simulink model "Copy_3_of_proba1_poziomywsk"  (Simulink 7.0)
settings: Solver=ode1  StartTime=0.0  StopTime=Inf  FixedStep=0.001  RelTol=1e-3
PostLoadFcn:
  | ,try, rti_mdl_postloadfcn(bdroot, 'UpdateModel', 280, 'rti1005'); catch, disp(lasterr); end,
values from neighbouring files (symbols this model uses):
  Rmax = 823    [50614_9.mat]
  Rmin = 331    [50614_9.mat]
undefined symbols (not defined in the file or in its folder): sgn
libraries: simulink x68, simulink_extras x15, rtilibm x10
(part 2 of 3)

== system Copy_3_of_proba1_poziomywsk/serwomechanizmy/os1/ograniczenie1 ==
  In1 : Inport
  Compare To Constant : simulink/Logic and Bit Operations/Compare To Constant  SystemSampleTime=-1  relop=<=  const=160  LogicOutDataTypeMode=boolean  ZeroCross=off
  Compare To Constant1 : simulink/Logic and Bit Operations/Compare To Constant  SystemSampleTime=-1  relop=>=  const=-160  LogicOutDataTypeMode=boolean  ZeroCross=off
  Constant1 : Constant  Value=0
  Logical Operator : Logic  AllPortsSameDT=off  OutDataTypeMode=boolean
  Switch : Switch  Criteria=u2 ~= 0
  Out1 : Outport
  wires:
  In1/1 -> Compare To Constant/1, Compare To Constant1/1, Switch/1
  Compare To Constant1/1 -> Logical Operator/1
  Compare To Constant/1 -> Logical Operator/2
  Logical Operator/1 -> Switch/2
  Constant1/1 -> Switch/3
  Switch/1 -> Out1/1

== system Copy_3_of_proba1_poziomywsk/serwomechanizmy/os2/Position 2 ==
  Sin && Cos2 : Inport
  Reset 2 : Inport  Port=2
  Filters 2 : Subsystem
  Position Calculation 2 : Subsystem
  Out1 : Outport
  wires:
  Filters 2/1(Sin) -> Position Calculation 2/1(Sin)
  Filters 2/2(Cos) -> Position Calculation 2/2(Cos)
  Sin && Cos2/1 -> Filters 2/1(Sin && Cos)
  Reset 2/1 -> Position Calculation 2/3(Reset (Impulse))
  Position Calculation 2/1(Position) -> Out1/1

== system Copy_3_of_proba1_poziomywsk/serwomechanizmy/os2/blok bazowania ==
  bazowanie : Inport
  stop : Inport  Port=2
  DS2201IN_B1 : rtilibm/DS2201/DS2201IN_B1  SystemSampleTime=-1  BoardNo=1  ChannelNos=2  DialogFcn=gui2201in  UnitName={ 'DS2201IN_B' }  UnitValues={ 1 }  DSProperties=struct('RTI',struct('Version',uint32(1),'BlockType',struct('isSLSource',uint8(1),'isSLSink',uint8(0),'isHWSource',uint8(1),'isHWSink',uint8(0),'isSetup',uint8(0),'isInline',uint8(1),'isNonInline',uint8(0),'isInterrupt',uint8(0),'isChannelwise',uint8(0)),'IOBoardType','DS2201','UnitType','BIT','Identifier','BITIN','DialogType','ML','BlockSet','NONE','SlaveProcessor','NONE'))
  Logical Operator : Logic  Operator=OR  AllPortsSameDT=off
  S-R Flip-Flop : simulink_extras/Flip Flops/S-R Flip-Flop  SystemSampleTime=-1  initial_condition=0
  zerowanie : Subsystem  TreatAsAtomicUnit=on
  reset : Outport
  bool : Outport  Port=2
  wires:
  bazowanie/1 -> S-R Flip-Flop/1
  S-R Flip-Flop/1 -> bool/1, zerowanie/Enable
  S-R Flip-Flop/2 -> reset/1
  stop/1 -> Logical Operator/2
  Logical Operator/1 -> S-R Flip-Flop/2
  DS2201IN_B1/1 -> Logical Operator/1

== system Copy_3_of_proba1_poziomywsk/serwomechanizmy/os2/blok stopu ==
  pozycja : Inport
  Trigger : TriggerPort
  Data Store Write : DataStoreWrite  DataStoreName=u2  SampleTime=-1
  Data Store Write1 : DataStoreWrite  DataStoreName=tmp_u2  SampleTime=-1
  wires:
  pozycja/1 -> Data Store Write/1, Data Store Write1/1

== system Copy_3_of_proba1_poziomywsk/serwomechanizmy/os2/ograniczenie2 ==
  In1 : Inport
  Compare To Constant : simulink/Logic and Bit Operations/Compare To Constant  SystemSampleTime=-1  relop=<=  const=40  LogicOutDataTypeMode=boolean  ZeroCross=off
  Compare To Constant1 : simulink/Logic and Bit Operations/Compare To Constant  SystemSampleTime=-1  relop=>=  const=-40  LogicOutDataTypeMode=boolean  ZeroCross=off
  Constant1 : Constant  Value=0
  Logical Operator : Logic  AllPortsSameDT=off  OutDataTypeMode=boolean
  Switch : Switch  Criteria=u2 ~= 0
  Out1 : Outport
  wires:
  In1/1 -> Compare To Constant/1, Compare To Constant1/1, Switch/1
  Compare To Constant1/1 -> Logical Operator/1
  Compare To Constant/1 -> Logical Operator/2
  Logical Operator/1 -> Switch/2
  Constant1/1 -> Switch/3
  Switch/1 -> Out1/1

== system Copy_3_of_proba1_poziomywsk/serwomechanizmy/os3/Position 3 ==
  Sin && Cos3 : Inport
  Reset 3 : Inport  Port=2
  Filters 3 : Subsystem
  Position Calculation 3 : Subsystem
  Out1 : Outport
  wires:
  Filters 3/1(Sin) -> Position Calculation 3/1(Sin)
  Filters 3/2(Cos) -> Position Calculation 3/2(Cos)
  Sin && Cos3/1 -> Filters 3/1(Sin && Cos)
  Reset 3/1 -> Position Calculation 3/3(Reset (Impulse))
  Position Calculation 3/1(Position) -> Out1/1

== system Copy_3_of_proba1_poziomywsk/serwomechanizmy/os3/blok bazowania ==
  bazowanie : Inport
  stop : Inport  Port=2
  DS2201IN_B1 : rtilibm/DS2201/DS2201IN_B1  SystemSampleTime=-1  BoardNo=1  ChannelNos=3  DialogFcn=gui2201in  UnitName={ 'DS2201IN_B' }  UnitValues={ 1 }  DSProperties=struct('RTI',struct('Version',uint32(1),'BlockType',struct('isSLSource',uint8(1),'isSLSink',uint8(0),'isHWSource',uint8(1),'isHWSink',uint8(0),'isSetup',uint8(0),'isInline',uint8(1),'isNonInline',uint8(0),'isInterrupt',uint8(0),'isChannelwise',uint8(0)),'IOBoardType','DS2201','UnitType','BIT','Identifier','BITIN','DialogType','ML','BlockSet','NONE','SlaveProcessor','NONE'))
  Logical Operator : Logic  Operator=OR  AllPortsSameDT=off
  S-R Flip-Flop : simulink_extras/Flip Flops/S-R Flip-Flop  SystemSampleTime=-1  initial_condition=0
  zerowanie : Subsystem  TreatAsAtomicUnit=on
  reset : Outport
  bool : Outport  Port=2
  wires:
  bazowanie/1 -> S-R Flip-Flop/1
  S-R Flip-Flop/1 -> bool/1, zerowanie/Enable
  S-R Flip-Flop/2 -> reset/1
  stop/1 -> Logical Operator/2
  DS2201IN_B1/1 -> Logical Operator/1
  Logical Operator/1 -> S-R Flip-Flop/2

== system Copy_3_of_proba1_poziomywsk/serwomechanizmy/os3/blok stopu ==
  pozycja : Inport
  Trigger : TriggerPort
  Data Store Write : DataStoreWrite  DataStoreName=u3  SampleTime=-1
  Data Store Write1 : DataStoreWrite  DataStoreName=tmp_u3  SampleTime=-1
  wires:
  pozycja/1 -> Data Store Write/1, Data Store Write1/1

== system Copy_3_of_proba1_poziomywsk/serwomechanizmy/os3/ograniczenie3 ==
  In1 : Inport
  Compare To Constant : simulink/Logic and Bit Operations/Compare To Constant  SystemSampleTime=-1  relop=<=  const=40  LogicOutDataTypeMode=boolean  ZeroCross=off
  Compare To Constant1 : simulink/Logic and Bit Operations/Compare To Constant  SystemSampleTime=-1  relop=>=  const=-25  LogicOutDataTypeMode=boolean  ZeroCross=off
  Constant1 : Constant  Value=0
  Logical Operator : Logic  AllPortsSameDT=off  OutDataTypeMode=boolean
  Switch : Switch  Criteria=u2 ~= 0
  Out1 : Outport
  wires:
  In1/1 -> Compare To Constant/1, Compare To Constant1/1, Switch/1
  Compare To Constant1/1 -> Logical Operator/1
  Compare To Constant/1 -> Logical Operator/2
  Logical Operator/1 -> Switch/2
  Constant1/1 -> Switch/3
  Switch/1 -> Out1/1

== system Copy_3_of_proba1_poziomywsk/serwomechanizmy/os4/Position 4 ==
  Sin && Cos4 : Inport
  Reset 4 : Inport  Port=2
  Filters 4 : Subsystem
  Position Calculation 4 : Subsystem
  Out1 : Outport
  wires:
  Position Calculation 4/1(Position) -> Out1/1
  Reset 4/1 -> Position Calculation 4/3(Reset (Impulse))
  Sin && Cos4/1 -> Filters 4/1(Sin && Cos)
  Filters 4/2(Cos) -> Position Calculation 4/2(Cos)
  Filters 4/1(Sin) -> Position Calculation 4/1(Sin)

== system Copy_3_of_proba1_poziomywsk/serwomechanizmy/os4/blok bazowania ==
  bazowanie : Inport
  stop : Inport  Port=2
  DS2201IN_B1 : rtilibm/DS2201/DS2201IN_B1  SystemSampleTime=-1  BoardNo=1  ChannelNos=4  DialogFcn=gui2201in  UnitName={ 'DS2201IN_B' }  UnitValues={ 1 }  DSProperties=struct('RTI',struct('Version',uint32(1),'BlockType',struct('isSLSource',uint8(1),'isSLSink',uint8(0),'isHWSource',uint8(1),'isHWSink',uint8(0),'isSetup',uint8(0),'isInline',uint8(1),'isNonInline',uint8(0),'isInterrupt',uint8(0),'isChannelwise',uint8(0)),'IOBoardType','DS2201','UnitType','BIT','Identifier','BITIN','DialogType','ML','BlockSet','NONE','SlaveProcessor','NONE'))
  Logical Operator : Logic  Operator=OR  AllPortsSameDT=off
  S-R Flip-Flop : simulink_extras/Flip Flops/S-R Flip-Flop  SystemSampleTime=-1  initial_condition=0
  zerowanie : Subsystem  TreatAsAtomicUnit=on
  reset : Outport
  bool : Outport  Port=2
  wires:
  bazowanie/1 -> S-R Flip-Flop/1
  S-R Flip-Flop/1 -> bool/1, zerowanie/Enable
  S-R Flip-Flop/2 -> reset/1
  stop/1 -> Logical Operator/2
  DS2201IN_B1/1 -> Logical Operator/1
  Logical Operator/1 -> S-R Flip-Flop/2

== system Copy_3_of_proba1_poziomywsk/serwomechanizmy/os4/blok stopu ==
  pozycja : Inport
  Trigger : TriggerPort
  Data Store Write : DataStoreWrite  DataStoreName=u4  SampleTime=-1
  Data Store Write1 : DataStoreWrite  DataStoreName=tmp_u4  SampleTime=-1
  wires:
  pozycja/1 -> Data Store Write/1, Data Store Write1/1

== system Copy_3_of_proba1_poziomywsk/serwomechanizmy/os4/ograniczenie3 ==
  In1 : Inport
  Compare To Constant : simulink/Logic and Bit Operations/Compare To Constant  SystemSampleTime=-1  relop=<=  const=120  LogicOutDataTypeMode=boolean  ZeroCross=off
  Compare To Constant1 : simulink/Logic and Bit Operations/Compare To Constant  SystemSampleTime=-1  relop=>=  const=-25  LogicOutDataTypeMode=boolean  ZeroCross=off
  Constant1 : Constant  Value=0
  Logical Operator : Logic  AllPortsSameDT=off  OutDataTypeMode=boolean
  Switch : Switch  Criteria=u2 ~= 0
  Out1 : Outport
  wires:
  In1/1 -> Compare To Constant/1, Compare To Constant1/1, Switch/1
  Compare To Constant1/1 -> Logical Operator/1
  Compare To Constant/1 -> Logical Operator/2
  Logical Operator/1 -> Switch/2
  Constant1/1 -> Switch/3
  Switch/1 -> Out1/1

== system Copy_3_of_proba1_poziomywsk/serwomechanizmy/os5/Position 5 ==
  Sin && Cos5 : Inport
  Reset 5 : Inport  Port=2
  Filters 5 : Subsystem
  Position Calculation 5 : Subsystem
  Out1 : Outport
  wires:
  Position Calculation 5/1(Position) -> Out1/1
  Reset 5/1 -> Position Calculation 5/3(Reset (Impulse))
  Sin && Cos5/1 -> Filters 5/1(Sin && Cos)
  Filters 5/2(Cos) -> Position Calculation 5/2(Cos)
  Filters 5/1(Sin) -> Position Calculation 5/1(Sin)

== system Copy_3_of_proba1_poziomywsk/serwomechanizmy/os5/blok bazowania ==
  bazowanie : Inport
  stop : Inport  Port=2
  DS2201IN_B1 : rtilibm/DS2201/DS2201IN_B1  SystemSampleTime=-1  BoardNo=1  ChannelNos=5  DialogFcn=gui2201in  UnitName={ 'DS2201IN_B' }  UnitValues={ 1 }  DSProperties=struct('RTI',struct('Version',uint32(1),'BlockType',struct('isSLSource',uint8(1),'isSLSink',uint8(0),'isHWSource',uint8(1),'isHWSink',uint8(0),'isSetup',uint8(0),'isInline',uint8(1),'isNonInline',uint8(0),'isInterrupt',uint8(0),'isChannelwise',uint8(0)),'IOBoardType','DS2201','UnitType','BIT','Identifier','BITIN','DialogType','ML','BlockSet','NONE','SlaveProcessor','NONE'))
  Logical Operator : Logic  Operator=OR  AllPortsSameDT=off
  S-R Flip-Flop : simulink_extras/Flip Flops/S-R Flip-Flop  SystemSampleTime=-1  initial_condition=0
  zerowanie : Subsystem  TreatAsAtomicUnit=on
  reset : Outport
  bool : Outport  Port=2
  wires:
  bazowanie/1 -> S-R Flip-Flop/1
  S-R Flip-Flop/1 -> bool/1, zerowanie/Enable
  S-R Flip-Flop/2 -> reset/1
  stop/1 -> Logical Operator/2
  DS2201IN_B1/1 -> Logical Operator/1
  Logical Operator/1 -> S-R Flip-Flop/2

== system Copy_3_of_proba1_poziomywsk/serwomechanizmy/os5/blok stopu ==
  pozycja : Inport
  Trigger : TriggerPort
  Data Store Write : DataStoreWrite  DataStoreName=u5  SampleTime=-1
  Data Store Write1 : DataStoreWrite  DataStoreName=tmp_u5  SampleTime=-1
  wires:
  pozycja/1 -> Data Store Write/1, Data Store Write1/1

== system Copy_3_of_proba1_poziomywsk/serwomechanizmy/os5/ograniczenie3 ==
  In1 : Inport
  Compare To Constant : simulink/Logic and Bit Operations/Compare To Constant  SystemSampleTime=-1  relop=<=  const=150  LogicOutDataTypeMode=boolean  ZeroCross=off
  Compare To Constant1 : simulink/Logic and Bit Operations/Compare To Constant  SystemSampleTime=-1  relop=>=  const=-25  LogicOutDataTypeMode=boolean  ZeroCross=off
  Constant1 : Constant  Value=0
  Logical Operator : Logic  AllPortsSameDT=off  OutDataTypeMode=boolean
  Switch : Switch  Criteria=u2 ~= 0
  Out1 : Outport
  wires:
  In1/1 -> Compare To Constant/1, Compare To Constant1/1, Switch/1
  Compare To Constant1/1 -> Logical Operator/1
  Compare To Constant/1 -> Logical Operator/2
  Logical Operator/1 -> Switch/2
  Constant1/1 -> Switch/3
  Switch/1 -> Out1/1

== system Copy_3_of_proba1_poziomywsk/serwomechanizmy/os6/blok bazowania ==
  bazowanie : Inport
  stop : Inport  Port=2
  DS2201IN_B1 : rtilibm/DS2201/DS2201IN_B1  SystemSampleTime=-1  BoardNo=1  ChannelNos=6  DialogFcn=gui2201in  UnitName={ 'DS2201IN_B' }  UnitValues={ 1 }  DSProperties=struct('RTI',struct('Version',uint32(1),'BlockType',struct('isSLSource',uint8(1),'isSLSink',uint8(0),'isHWSource',uint8(1),'isHWSink',uint8(0),'isSetup',uint8(0),'isInline',uint8(1),'isNonInline',uint8(0),'isInterrupt',uint8(0),'isChannelwise',uint8(0)),'IOBoardType','DS2201','UnitType','BIT','Identifier','BITIN','DialogType','ML','BlockSet','NONE','SlaveProcessor','NONE'))
  Logical Operator : Logic  Operator=OR  AllPortsSameDT=off
  S-R Flip-Flop : simulink_extras/Flip Flops/S-R Flip-Flop  SystemSampleTime=-1  initial_condition=0
  zerowanie : Subsystem  TreatAsAtomicUnit=on
  reset : Outport
  bool : Outport  Port=2
  wires:
  bazowanie/1 -> S-R Flip-Flop/1
  S-R Flip-Flop/1 -> bool/1, zerowanie/Enable
  S-R Flip-Flop/2 -> reset/1
  stop/1 -> Logical Operator/2
  DS2201IN_B1/1 -> Logical Operator/1
  Logical Operator/1 -> S-R Flip-Flop/2

== system Copy_3_of_proba1_poziomywsk/serwomechanizmy/os6/blok stopu ==
  pozycja : Inport
  Trigger : TriggerPort
  Data Store Write : DataStoreWrite  DataStoreName=u0  SampleTime=-1
  Data Store Write1 : DataStoreWrite  DataStoreName=tmp_u0  SampleTime=-1
  wires:
  pozycja/1 -> Data Store Write/1, Data Store Write1/1

== system Copy_3_of_proba1_poziomywsk/serwomechanizmy/os6/ograniczenie3 ==
  In1 : Inport
  Compare To Constant : simulink/Logic and Bit Operations/Compare To Constant  SystemSampleTime=-1  relop=<=  const=890  LogicOutDataTypeMode=boolean  ZeroCross=off
  Compare To Constant1 : simulink/Logic and Bit Operations/Compare To Constant  SystemSampleTime=-1  relop=>=  const=0  LogicOutDataTypeMode=boolean  ZeroCross=off
  Constant1 : Constant  Value=0
  Logical Operator : Logic  AllPortsSameDT=off  OutDataTypeMode=boolean
  Switch : Switch  Criteria=u2 ~= 0
  Out1 : Outport
  wires:
  In1/1 -> Compare To Constant/1, Compare To Constant1/1, Switch/1
  Compare To Constant1/1 -> Logical Operator/1
  Compare To Constant/1 -> Logical Operator/2
  Logical Operator/1 -> Switch/2
  Constant1/1 -> Switch/3
  Switch/1 -> Out1/1

== system Copy_3_of_proba1_poziomywsk/serwomechanizmy/os6/skalowanie ==
  In1 : Inport
  Fcn : Fcn  Expr=(u(1)*(2^23)*pi())/1000
  Gain2 : Gain  Gain=1.25/pi()
  Out1 : Outport
  wires:
  Fcn/1 -> Gain2/1
  Gain2/1 -> Out1/1
  In1/1 -> Fcn/1

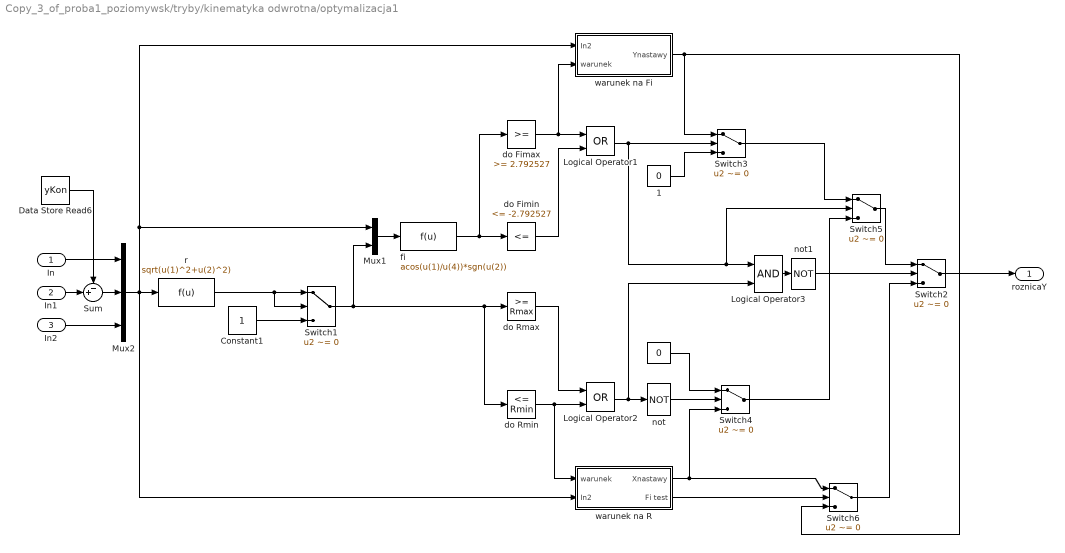
== system Copy_3_of_proba1_poziomywsk/tryby/kinematyka odwrotna/optymalizacja1 ==
  In : Inport
  In1 : Inport  Port=2
  In2 : Inport  Port=3
  " " : Constant  Value=0  OutDataTypeMode=double
  " 1" : Constant  Value=0  OutDataTypeMode=double
  Constant1 : Constant  OutDataTypeMode=double
  Data Store Read6 : DataStoreRead  DataStoreName=yKon  SampleTime=0
  Logical Operator1 : Logic  Operator=OR  AllPortsSameDT=off  OutDataTypeMode=boolean
  Logical Operator2 : Logic  Operator=OR  AllPortsSameDT=off  OutDataTypeMode=boolean
  Logical Operator3 : Logic  AllPortsSameDT=off  OutDataTypeMode=boolean
  Mux1 : Mux  Inputs=2
  Mux2 : Mux  Inputs=3
  Sum : Sum  Inputs=-+|
  Switch1 : Switch  Criteria=u2 ~= 0  OutDataTypeMode=double
  Switch{2..6} (5 alike) : Switch  Criteria=u2 ~= 0
  do Fimax : simulink/Logic and Bit Operations/Compare To Constant  SystemSampleTime=-1  relop=>=  const=2.792527  LogicOutDataTypeMode=uint8  ZeroCross=off
  do Fimin : simulink/Logic and Bit Operations/Compare To Constant  SystemSampleTime=-1  relop=<=  const=-2.792527  LogicOutDataTypeMode=uint8  ZeroCross=off
  do Rmax : simulink/Logic and Bit Operations/Compare To Constant  SystemSampleTime=-1  relop=>=  const=Rmax  LogicOutDataTypeMode=uint8  ZeroCross=off
  do Rmin : simulink/Logic and Bit Operations/Compare To Constant  SystemSampleTime=-1  relop=<=  const=Rmin  LogicOutDataTypeMode=uint8  ZeroCross=off
  fi : Fcn  Expr=acos(u(1)/u(4))*sgn(u(2))
  not : Logic  Operator=NOT  AllPortsSameDT=off  OutDataTypeMode=boolean
  not1 : Logic  Operator=NOT  AllPortsSameDT=off  OutDataTypeMode=boolean
  r : Fcn  Expr=sqrt(u(1)^2+u(2)^2)
  warunek na Fi : Subsystem  TreatAsAtomicUnit=on
  warunek na R : Subsystem  TreatAsAtomicUnit=on
  roznicaY : Outport
  wires:
  Switch6/1 -> Switch2/3
  warunek na R/2(Fi test) -> Switch6/2
  not1/1 -> Switch2/2
  Switch3/1 -> Switch5/1
  Switch4/1 -> Switch5/3
  Switch5/1 -> Switch2/1
  Logical Operator3/1 -> not1/1
  " 1"/1 -> Switch3/3
  " "/1 -> Switch4/1
  not/1 -> Switch4/2
  warunek na R/1(Xnastawy) -> Switch4/3, Switch6/1
  warunek na Fi/1(Ynastawy) -> Switch3/1, Switch6/3
  Logical Operator1/1 -> Switch3/2, Logical Operator3/1, Switch5/2
  Logical Operator2/1 -> not/1, Logical Operator3/2
  do Rmin/1 -> Logical Operator2/2, warunek na R/1(warunek)
  do Rmax/1 -> Logical Operator2/1
  do Fimin/1 -> Logical Operator1/2
  do Fimax/1 -> warunek na Fi/2(warunek), Logical Operator1/1
  fi/1 -> do Fimin/1, do Fimax/1
  Constant1/1 -> Switch1/3
  Mux1/1 -> fi/1
  Switch1/1 -> Mux1/2, do Rmax/1, do Rmin/1
  r/1 -> Switch1/2, Switch1/1
  Mux2/1 -> r/1, Mux1/1, warunek na Fi/1(In2), warunek na R/2(In2)
  In/1 -> Mux2/1
  In2/1 -> Mux2/3
  Switch2/1 -> roznicaY/1
  Sum/1 -> Mux2/2
  In1/1 -> Sum/2
  Data Store Read6/1 -> Sum/1

== system Copy_3_of_proba1_poziomywsk/tryby/kinematyka odwrotna/podaj wyliczone wartosci ==
  obliczoneFi1 : Inport
  obliczoneFi2 : Inport  Port=2
  obliczoneFi3 : Inport  Port=3
  obliczoneDist : Inport  Port=4
  Enable : EnablePort
  Data Store Write : DataStoreWrite  DataStoreName=obliczoneFi1  SampleTime=-1
  Data Store Write1 : DataStoreWrite  DataStoreName=obliczoneFi2  SampleTime=-1
  Data Store Write2 : DataStoreWrite  DataStoreName=obliczoneFi3  SampleTime=-1
  Data Store Write3 : DataStoreWrite  DataStoreName=obliczoneDist  SampleTime=-1
  wires:
  obliczoneFi1/1 -> Data Store Write/1
  obliczoneFi2/1 -> Data Store Write1/1
  obliczoneFi3/1 -> Data Store Write2/1
  obliczoneDist/1 -> Data Store Write3/1

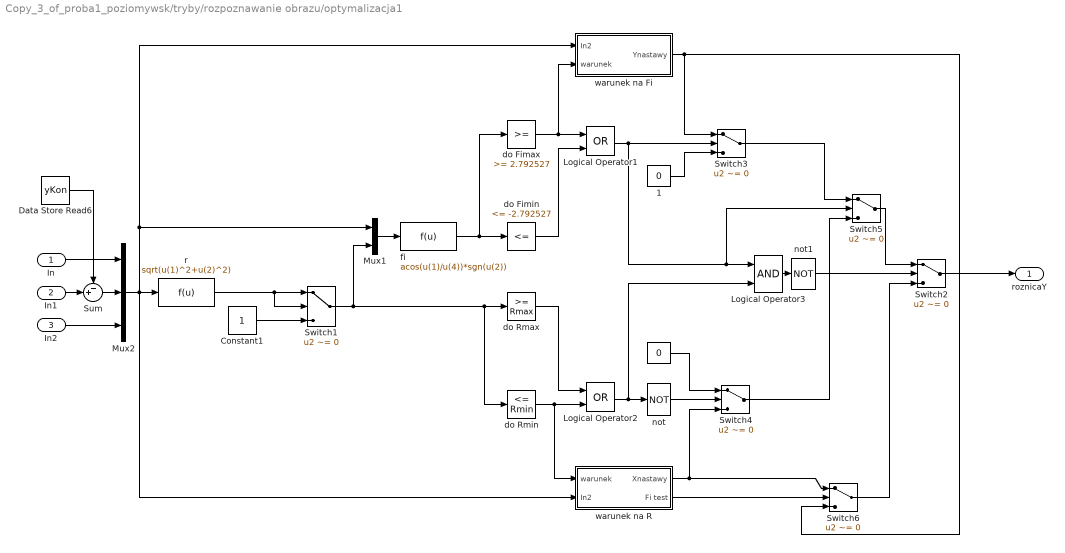
== system Copy_3_of_proba1_poziomywsk/tryby/rozpoznawanie obrazu/optymalizacja1 ==
  In : Inport
  In1 : Inport  Port=2
  In2 : Inport  Port=3
  " " : Constant  Value=0  OutDataTypeMode=double
  " 1" : Constant  Value=0  OutDataTypeMode=double
  Constant1 : Constant  OutDataTypeMode=double
  Data Store Read6 : DataStoreRead  DataStoreName=yKon  SampleTime=-1
  Logical Operator1 : Logic  Operator=OR  AllPortsSameDT=off  OutDataTypeMode=boolean
  Logical Operator2 : Logic  Operator=OR  AllPortsSameDT=off  OutDataTypeMode=boolean
  Logical Operator3 : Logic  AllPortsSameDT=off  OutDataTypeMode=boolean
  Mux1 : Mux  Inputs=2
  Mux2 : Mux  Inputs=3
  Sum : Sum  Inputs=-+|
  Switch1 : Switch  Criteria=u2 ~= 0  OutDataTypeMode=double
  Switch{2..6} (5 alike) : Switch  Criteria=u2 ~= 0
  do Fimax : simulink/Logic and Bit Operations/Compare To Constant  SystemSampleTime=-1  relop=>=  const=2.792527  LogicOutDataTypeMode=uint8  ZeroCross=off
  do Fimin : simulink/Logic and Bit Operations/Compare To Constant  SystemSampleTime=-1  relop=<=  const=-2.792527  LogicOutDataTypeMode=uint8  ZeroCross=off
  do Rmax : simulink/Logic and Bit Operations/Compare To Constant  SystemSampleTime=-1  relop=>=  const=Rmax  LogicOutDataTypeMode=uint8  ZeroCross=off
  do Rmin : simulink/Logic and Bit Operations/Compare To Constant  SystemSampleTime=-1  relop=<=  const=Rmin  LogicOutDataTypeMode=uint8  ZeroCross=off
  fi : Fcn  Expr=acos(u(1)/u(4))*sgn(u(2))
  not : Logic  Operator=NOT  AllPortsSameDT=off  OutDataTypeMode=boolean
  not1 : Logic  Operator=NOT  AllPortsSameDT=off  OutDataTypeMode=boolean
  r : Fcn  Expr=sqrt(u(1)^2+u(2)^2)
  warunek na Fi : Subsystem  TreatAsAtomicUnit=on
  warunek na R : Subsystem  TreatAsAtomicUnit=on
  roznicaY : Outport
  wires:
  Data Store Read6/1 -> Sum/1
  In1/1 -> Sum/2
  Sum/1 -> Mux2/2
  Switch2/1 -> roznicaY/1
  In2/1 -> Mux2/3
  In/1 -> Mux2/1
  Mux2/1 -> warunek na R/2(In2), warunek na Fi/1(In2), Mux1/1, r/1
  r/1 -> Switch1/1, Switch1/2
  Switch1/1 -> do Rmin/1, do Rmax/1, Mux1/2
  Mux1/1 -> fi/1
  Constant1/1 -> Switch1/3
  fi/1 -> do Fimax/1, do Fimin/1
  do Fimax/1 -> Logical Operator1/1, warunek na Fi/2(warunek)
  do Fimin/1 -> Logical Operator1/2
  do Rmax/1 -> Logical Operator2/1
  do Rmin/1 -> warunek na R/1(warunek), Logical Operator2/2
  Logical Operator2/1 -> Logical Operator3/2, not/1
  Logical Operator1/1 -> Switch5/2, Logical Operator3/1, Switch3/2
  warunek na Fi/1(Ynastawy) -> Switch6/3, Switch3/1
  warunek na R/1(Xnastawy) -> Switch6/1, Switch4/3
  not/1 -> Switch4/2
  " "/1 -> Switch4/1
  " 1"/1 -> Switch3/3
  Logical Operator3/1 -> not1/1
  Switch5/1 -> Switch2/1
  Switch4/1 -> Switch5/3
  Switch3/1 -> Switch5/1
  not1/1 -> Switch2/2
  warunek na R/2(Fi test) -> Switch6/2
  Switch6/1 -> Switch2/3

== system Copy_3_of_proba1_poziomywsk/tryby/rozpoznawanie obrazu/podaj wyliczone wartosci ==
  obliczoneFi1 : Inport
  obliczoneFi2 : Inport  Port=2
  obliczoneFi3 : Inport  Port=3
  obliczoneDist : Inport  Port=4
  Enable : EnablePort
  Data Store Write : DataStoreWrite  DataStoreName=obliczoneFi1  SampleTime=-1
  Data Store Write1 : DataStoreWrite  DataStoreName=obliczoneFi2  SampleTime=-1
  Data Store Write2 : DataStoreWrite  DataStoreName=obliczoneFi3  SampleTime=-1
  Data Store Write3 : DataStoreWrite  DataStoreName=obliczoneDist  SampleTime=-1
  wires:
  obliczoneDist/1 -> Data Store Write3/1
  obliczoneFi3/1 -> Data Store Write2/1
  obliczoneFi2/1 -> Data Store Write1/1
  obliczoneFi1/1 -> Data Store Write/1

== system Copy_3_of_proba1_poziomywsk/RTI Data/RTI Data Store/RTI Data Store/RTI Data Store ==
  RTI Data Store : Subsystem
      mask Type: RTI_DATA_STORE
      mask Description:
      | RTI Data Store Block. This block is used by RTI to store internal model dependent data. Deleting this block will result in data loss.
      | 
      | NEVER DELETE, COPY, OR MODIFY THIS BLOCK!
      mask Help:
      | RTI Data Store Block. This block is used by RTI to store internal model dependent data. Deleting this block will result in data loss.
      | 
      | NEVER DELETE, COPY, OR MODIFY THIS BLOCK!
      mask Display: text(0.5, 0.5, ' ', 'HorizontalAlignment', 'center');

== system Copy_3_of_proba1_poziomywsk/serwomechanizmy/os1/Position 1/Filters 1 ==
  Sin && Cos : Inport
  Analog Butterworth LP Filter : Subsystem  mask(buttap){@1=2*pi*16, @2=1}
      mask prompts: @1 "Cutoff frequency (rad/sec)"; @2 "Order"
      mask help:
      | Analog Butterworth low pass filter.
      |
      | (Requires Signal Processing Toolbox)
      mask init:
      | [z,p,k]=buttap(@2); z=@1*z; p=@1*p; k=real(prod(-p)); [num,den]=zp2tf(z,p,k); w=logspace(log10(@1/10),log10(10*@1),20); h=freqs(num,den,w);
      mask Help: Butterworth low pass filter using MATLAB's butter command.
      mask Display: plot(20*log10(w),20*log10(abs(h)))
  Analog Butterworth LP Filter1 : Subsystem  mask(buttap){@1=2*pi*16, @2=1}
      mask prompts: @1 "Cutoff frequency (rad/sec)"; @2 "Order"
      mask help:
      | Analog Butterworth low pass filter.
      |
      | (Requires Signal Processing Toolbox)
      mask init:
      | [z,p,k]=buttap(@2); z=@1*z; p=@1*p; k=real(prod(-p)); [num,den]=zp2tf(z,p,k); w=logspace(log10(@1/10),log10(10*@1),20); h=freqs(num,den,w);
      mask Help: Butterworth low pass filter using MATLAB's butter command.
      mask Display: plot(20*log10(w),20*log10(abs(h)))
  Demux : Demux  Outputs=2
  Sin : Outport
  Cos : Outport  Port=2
  wires:
  Demux/2 -> Analog Butterworth LP Filter1/1(In1)
  Demux/1 -> Analog Butterworth LP Filter/1(In1)
  Sin && Cos/1 -> Demux/1
  Analog Butterworth LP Filter1/1(Out1) -> Cos/1
  Analog Butterworth LP Filter/1(Out1) -> Sin/1

== system Copy_3_of_proba1_poziomywsk/serwomechanizmy/os1/Position 1/Position Calculation 1 ==
  Sin : Inport
  Cos : Inport  Port=2
  Reset (Impulse) : Inport  Port=3
  Atan2 : Fcn  Expr=atan2(u[1],u[2])
  Conversion Rad to Deg : Gain  Gain=180/pi  SaturateOnIntegerOverflow=on
  Conversion Rotation to Angle : Gain  Gain=2*pi  SaturateOnIntegerOverflow=on
  Dead Zone : DeadZone  LowerValue=-5000  UpperValue=5000  SaturateOnIntegerOverflow=on
  Derivative : Derivative
  Gear : Gain  Gain=6.33e-3  SaturateOnIntegerOverflow=on
  Init Angle : Switch  Threshold=1  SaturateOnIntegerOverflow=on  InputSameDT=on
  Memory : Memory  Orientation=left
  Memory1 : Memory  Orientation=left
  Mux : Mux  Inputs=2
  Product : Product  SaturateOnIntegerOverflow=on  RndMeth=Zero  InputSameDT=on
  Saturation : Saturate  UpperLimit=1  LowerLimit=-1
  Sum : Sum  Inputs=+-  SaturateOnIntegerOverflow=on  InputSameDT=on
  Sum1 : Sum  Inputs=++-  SaturateOnIntegerOverflow=on  InputSameDT=on
  Position : Outport
  wires:
  Init Angle/1 -> Memory1/1, Sum1/3
  Memory1/1 -> Init Angle/1
  Product/1 -> Memory/1, Conversion Rotation to Angle/1
  Memory/1 -> Sum/1
  Cos/1 -> Mux/2
  Atan2/1 -> Init Angle/3, Sum1/2, Derivative/1
  Reset (Impulse)/1 -> Init Angle/2, Product/2
  Conversion Rotation to Angle/1 -> Sum1/1
  Saturation/1 -> Sum/2
  Conversion Rad to Deg/1 -> Position/1
  Sin/1 -> Mux/1
  Mux/1 -> Atan2/1
  Derivative/1 -> Dead Zone/1
  Dead Zone/1 -> Saturation/1
  Sum/1 -> Product/1
  Sum1/1 -> Gear/1
  Gear/1 -> Conversion Rad to Deg/1

== system Copy_3_of_proba1_poziomywsk/serwomechanizmy/os1/blok bazowania/zerowanie ==
  Enable : EnablePort
  Constant : Constant  Value=0
  Data Store Write : DataStoreWrite  DataStoreName=u1  SampleTime=-1
  Data Store Write1 : DataStoreWrite  DataStoreName=tmp_u1  SampleTime=-1
  wires:
  Constant/1 -> Data Store Write/1, Data Store Write1/1

== system Copy_3_of_proba1_poziomywsk/serwomechanizmy/os2/Position 2/Filters 2 ==
  Sin && Cos : Inport
  Analog Butterworth LP Filter : Subsystem  mask(buttap){@1=2*pi*16, @2=1}
      mask prompts: @1 "Cutoff frequency (rad/sec)"; @2 "Order"
      mask help:
      | Analog Butterworth low pass filter.
      |
      | (Requires Signal Processing Toolbox)
      mask init:
      | [z,p,k]=buttap(@2); z=@1*z; p=@1*p; k=real(prod(-p)); [num,den]=zp2tf(z,p,k); w=logspace(log10(@1/10),log10(10*@1),20); h=freqs(num,den,w);
      mask Help: Butterworth low pass filter using MATLAB's butter command.
      mask Display: plot(20*log10(w),20*log10(abs(h)))
  Analog Butterworth LP Filter1 : Subsystem  mask(buttap){@1=2*pi*16, @2=1}
      mask prompts: @1 "Cutoff frequency (rad/sec)"; @2 "Order"
      mask help:
      | Analog Butterworth low pass filter.
      |
      | (Requires Signal Processing Toolbox)
      mask init:
      | [z,p,k]=buttap(@2); z=@1*z; p=@1*p; k=real(prod(-p)); [num,den]=zp2tf(z,p,k); w=logspace(log10(@1/10),log10(10*@1),20); h=freqs(num,den,w);
      mask Help: Butterworth low pass filter using MATLAB's butter command.
      mask Display: plot(20*log10(w),20*log10(abs(h)))
  Demux : Demux  Outputs=2
  Sin : Outport
  Cos : Outport  Port=2
  wires:
  Demux/2 -> Analog Butterworth LP Filter1/1(In1)
  Demux/1 -> Analog Butterworth LP Filter/1(In1)
  Sin && Cos/1 -> Demux/1
  Analog Butterworth LP Filter1/1(Out1) -> Cos/1
  Analog Butterworth LP Filter/1(Out1) -> Sin/1

== system Copy_3_of_proba1_poziomywsk/serwomechanizmy/os2/Position 2/Position Calculation 2 ==
  Sin : Inport
  Cos : Inport  Port=2
  Reset (Impulse) : Inport  Port=3
  Atan2 : Fcn  Expr=atan2(u[1],u[2])
  Conversion Rad to Deg : Gain  Gain=180/pi  SaturateOnIntegerOverflow=on
  Conversion Rotation to Angle : Gain  Gain=2*pi  SaturateOnIntegerOverflow=on
  Dead Zone : DeadZone  LowerValue=-5000  UpperValue=5000  SaturateOnIntegerOverflow=on
  Derivative : Derivative
  Gear : Gain  Gain=6.37e-3  SaturateOnIntegerOverflow=on
  Init Angle : Switch  Threshold=1  SaturateOnIntegerOverflow=on  InputSameDT=on
  Memory : Memory  Orientation=left
  Memory1 : Memory  Orientation=left
  Mux : Mux  Inputs=2
  Product : Product  SaturateOnIntegerOverflow=on  RndMeth=Zero  InputSameDT=on
  Saturation : Saturate  UpperLimit=1  LowerLimit=-1
  Sum : Sum  Inputs=+-  SaturateOnIntegerOverflow=on  InputSameDT=on
  Sum1 : Sum  Inputs=++-  SaturateOnIntegerOverflow=on  InputSameDT=on
  Position : Outport
  wires:
  Init Angle/1 -> Memory1/1, Sum1/3
  Memory1/1 -> Init Angle/1
  Product/1 -> Memory/1, Conversion Rotation to Angle/1
  Memory/1 -> Sum/1
  Cos/1 -> Mux/2
  Atan2/1 -> Init Angle/3, Sum1/2, Derivative/1
  Reset (Impulse)/1 -> Init Angle/2, Product/2
  Conversion Rotation to Angle/1 -> Sum1/1
  Saturation/1 -> Sum/2
  Conversion Rad to Deg/1 -> Position/1
  Sin/1 -> Mux/1
  Mux/1 -> Atan2/1
  Derivative/1 -> Dead Zone/1
  Dead Zone/1 -> Saturation/1
  Sum/1 -> Product/1
  Sum1/1 -> Gear/1
  Gear/1 -> Conversion Rad to Deg/1

== system Copy_3_of_proba1_poziomywsk/serwomechanizmy/os2/blok bazowania/zerowanie ==
  Enable : EnablePort
  Constant : Constant  Value=0
  Data Store Write : DataStoreWrite  DataStoreName=u2  SampleTime=-1
  Data Store Write1 : DataStoreWrite  DataStoreName=tmp_u2  SampleTime=-1
  wires:
  Constant/1 -> Data Store Write/1, Data Store Write1/1

== system Copy_3_of_proba1_poziomywsk/serwomechanizmy/os3/Position 3/Filters 3 ==
  Sin && Cos : Inport
  Analog Butterworth LP Filter : Subsystem  mask(buttap){@1=2*pi*16, @2=1}
      mask prompts: @1 "Cutoff frequency (rad/sec)"; @2 "Order"
      mask help:
      | Analog Butterworth low pass filter.
      |
      | (Requires Signal Processing Toolbox)
      mask init:
      | [z,p,k]=buttap(@2); z=@1*z; p=@1*p; k=real(prod(-p)); [num,den]=zp2tf(z,p,k); w=logspace(log10(@1/10),log10(10*@1),20); h=freqs(num,den,w);
      mask Help: Butterworth low pass filter using MATLAB's butter command.
      mask Display: plot(20*log10(w),20*log10(abs(h)))
  Analog Butterworth LP Filter1 : Subsystem  mask(buttap){@1=2*pi*16, @2=1}
      mask prompts: @1 "Cutoff frequency (rad/sec)"; @2 "Order"
      mask help:
      | Analog Butterworth low pass filter.
      |
      | (Requires Signal Processing Toolbox)
      mask init:
      | [z,p,k]=buttap(@2); z=@1*z; p=@1*p; k=real(prod(-p)); [num,den]=zp2tf(z,p,k); w=logspace(log10(@1/10),log10(10*@1),20); h=freqs(num,den,w);
      mask Help: Butterworth low pass filter using MATLAB's butter command.
      mask Display: plot(20*log10(w),20*log10(abs(h)))
  Demux : Demux  Outputs=2
  Sin : Outport
  Cos : Outport  Port=2
  wires:
  Demux/2 -> Analog Butterworth LP Filter1/1(In1)
  Demux/1 -> Analog Butterworth LP Filter/1(In1)
  Sin && Cos/1 -> Demux/1
  Analog Butterworth LP Filter1/1(Out1) -> Cos/1
  Analog Butterworth LP Filter/1(Out1) -> Sin/1

== system Copy_3_of_proba1_poziomywsk/serwomechanizmy/os3/Position 3/Position Calculation 3 ==
  Sin : Inport
  Cos : Inport  Port=2
  Reset (Impulse) : Inport  Port=3
  Atan2 : Fcn  Expr=atan2(u[1],u[2])
  Conversion Rad to Deg : Gain  Gain=180/pi  SaturateOnIntegerOverflow=on
  Conversion Rotation to Angle : Gain  Gain=2*pi  SaturateOnIntegerOverflow=on
  Dead Zone : DeadZone  LowerValue=-5000  UpperValue=5000  SaturateOnIntegerOverflow=on
  Derivative : Derivative
  Gear : Gain  Gain=6.33e-3  SaturateOnIntegerOverflow=on
  Init Angle : Switch  Threshold=1  SaturateOnIntegerOverflow=on  InputSameDT=on
  Memory : Memory  Orientation=left
  Memory1 : Memory  Orientation=left
  Mux : Mux  Inputs=2
  Product : Product  SaturateOnIntegerOverflow=on  RndMeth=Zero  InputSameDT=on
  Saturation : Saturate  UpperLimit=1  LowerLimit=-1
  Sum : Sum  Inputs=+-  SaturateOnIntegerOverflow=on  InputSameDT=on
  Sum1 : Sum  Inputs=++-  SaturateOnIntegerOverflow=on  InputSameDT=on
  Position : Outport
  wires:
  Init Angle/1 -> Memory1/1, Sum1/3
  Memory1/1 -> Init Angle/1
  Product/1 -> Memory/1, Conversion Rotation to Angle/1
  Memory/1 -> Sum/1
  Cos/1 -> Mux/2
  Atan2/1 -> Init Angle/3, Sum1/2, Derivative/1
  Reset (Impulse)/1 -> Init Angle/2, Product/2
  Conversion Rotation to Angle/1 -> Sum1/1
  Saturation/1 -> Sum/2
  Conversion Rad to Deg/1 -> Position/1
  Sin/1 -> Mux/1
  Mux/1 -> Atan2/1
  Derivative/1 -> Dead Zone/1
  Dead Zone/1 -> Saturation/1
  Sum/1 -> Product/1
  Sum1/1 -> Gear/1
  Gear/1 -> Conversion Rad to Deg/1

== system Copy_3_of_proba1_poziomywsk/serwomechanizmy/os3/blok bazowania/zerowanie ==
  Enable : EnablePort
  Constant : Constant  Value=0
  Data Store Write : DataStoreWrite  DataStoreName=u3  SampleTime=-1
  Data Store Write1 : DataStoreWrite  DataStoreName=tmp_u3  SampleTime=-1
  wires:
  Constant/1 -> Data Store Write/1, Data Store Write1/1

== system Copy_3_of_proba1_poziomywsk/serwomechanizmy/os4/Position 4/Filters 4 ==
  Sin && Cos : Inport
  Analog Butterworth LP Filter : Subsystem  mask(buttap){@1=2*pi*16, @2=1}
      mask prompts: @1 "Cutoff frequency (rad/sec)"; @2 "Order"
      mask help:
      | Analog Butterworth low pass filter.
      |
      | (Requires Signal Processing Toolbox)
      mask init:
      | [z,p,k]=buttap(@2); z=@1*z; p=@1*p; k=real(prod(-p)); [num,den]=zp2tf(z,p,k); w=logspace(log10(@1/10),log10(10*@1),20); h=freqs(num,den,w);
      mask Help: Butterworth low pass filter using MATLAB's butter command.
      mask Display: plot(20*log10(w),20*log10(abs(h)))
  Analog Butterworth LP Filter1 : Subsystem  mask(buttap){@1=2*pi*16, @2=1}
      mask prompts: @1 "Cutoff frequency (rad/sec)"; @2 "Order"
      mask help:
      | Analog Butterworth low pass filter.
      |
      | (Requires Signal Processing Toolbox)
      mask init:
      | [z,p,k]=buttap(@2); z=@1*z; p=@1*p; k=real(prod(-p)); [num,den]=zp2tf(z,p,k); w=logspace(log10(@1/10),log10(10*@1),20); h=freqs(num,den,w);
      mask Help: Butterworth low pass filter using MATLAB's butter command.
      mask Display: plot(20*log10(w),20*log10(abs(h)))
  Demux : Demux  Outputs=2
  Sin : Outport
  Cos : Outport  Port=2
  wires:
  Analog Butterworth LP Filter/1(Out1) -> Sin/1
  Analog Butterworth LP Filter1/1(Out1) -> Cos/1
  Sin && Cos/1 -> Demux/1
  Demux/1 -> Analog Butterworth LP Filter/1(In1)
  Demux/2 -> Analog Butterworth LP Filter1/1(In1)

== system Copy_3_of_proba1_poziomywsk/serwomechanizmy/os4/Position 4/Position Calculation 4 ==
  Sin : Inport
  Cos : Inport  Port=2
  Reset (Impulse) : Inport  Port=3
  Atan2 : Fcn  Expr=atan2(u[1],u[2])
  Conversion Rad to Deg : Gain  Gain=180/pi  SaturateOnIntegerOverflow=on
  Conversion Rotation to Angle : Gain  Gain=2*pi  SaturateOnIntegerOverflow=on
  Dead Zone : DeadZone  LowerValue=-5000  UpperValue=5000  SaturateOnIntegerOverflow=on
  Derivative : Derivative
  Gear : Gain  Gain=7.87e-3  SaturateOnIntegerOverflow=on
  Init Angle : Switch  Threshold=1  SaturateOnIntegerOverflow=on  InputSameDT=on
  Memory : Memory  Orientation=left
  Memory1 : Memory  Orientation=left
  Mux : Mux  Inputs=2
  Product : Product  SaturateOnIntegerOverflow=on  RndMeth=Zero  InputSameDT=on
  Saturation : Saturate  UpperLimit=1  LowerLimit=-1
  Sum : Sum  Inputs=+-  SaturateOnIntegerOverflow=on  InputSameDT=on
  Sum1 : Sum  Inputs=++-  SaturateOnIntegerOverflow=on  InputSameDT=on
  Position : Outport
  wires:
  Gear/1 -> Conversion Rad to Deg/1
  Sum1/1 -> Gear/1
  Sum/1 -> Product/1
  Dead Zone/1 -> Saturation/1
  Derivative/1 -> Dead Zone/1
  Mux/1 -> Atan2/1
  Sin/1 -> Mux/1
  Conversion Rad to Deg/1 -> Position/1
  Saturation/1 -> Sum/2
  Conversion Rotation to Angle/1 -> Sum1/1
  Reset (Impulse)/1 -> Product/2, Init Angle/2
  Atan2/1 -> Derivative/1, Sum1/2, Init Angle/3
  Cos/1 -> Mux/2
  Memory/1 -> Sum/1
  Product/1 -> Conversion Rotation to Angle/1, Memory/1
  Memory1/1 -> Init Angle/1
  Init Angle/1 -> Sum1/3, Memory1/1

== system Copy_3_of_proba1_poziomywsk/serwomechanizmy/os4/blok bazowania/zerowanie ==
  Enable : EnablePort
  Constant : Constant  Value=0
  Data Store Write : DataStoreWrite  DataStoreName=u4  SampleTime=-1
  Data Store Write1 : DataStoreWrite  DataStoreName=tmp_u4  SampleTime=-1
  wires:
  Constant/1 -> Data Store Write/1, Data Store Write1/1

== system Copy_3_of_proba1_poziomywsk/serwomechanizmy/os5/Position 5/Filters 5 ==
  Sin && Cos : Inport
  Analog Butterworth LP Filter : Subsystem  mask(buttap){@1=2*pi*16, @2=1}
      mask prompts: @1 "Cutoff frequency (rad/sec)"; @2 "Order"
      mask help:
      | Analog Butterworth low pass filter.
      |
      | (Requires Signal Processing Toolbox)
      mask init:
      | [z,p,k]=buttap(@2); z=@1*z; p=@1*p; k=real(prod(-p)); [num,den]=zp2tf(z,p,k); w=logspace(log10(@1/10),log10(10*@1),20); h=freqs(num,den,w);
      mask Help: Butterworth low pass filter using MATLAB's butter command.
      mask Display: plot(20*log10(w),20*log10(abs(h)))
  Analog Butterworth LP Filter1 : Subsystem  mask(buttap){@1=2*pi*16, @2=1}
      mask prompts: @1 "Cutoff frequency (rad/sec)"; @2 "Order"
      mask help:
      | Analog Butterworth low pass filter.
      |
      | (Requires Signal Processing Toolbox)
      mask init:
      | [z,p,k]=buttap(@2); z=@1*z; p=@1*p; k=real(prod(-p)); [num,den]=zp2tf(z,p,k); w=logspace(log10(@1/10),log10(10*@1),20); h=freqs(num,den,w);
      mask Help: Butterworth low pass filter using MATLAB's butter command.
      mask Display: plot(20*log10(w),20*log10(abs(h)))
  Demux : Demux  Outputs=2
  Sin : Outport
  Cos : Outport  Port=2
  wires:
  Analog Butterworth LP Filter/1(Out1) -> Sin/1
  Analog Butterworth LP Filter1/1(Out1) -> Cos/1
  Sin && Cos/1 -> Demux/1
  Demux/1 -> Analog Butterworth LP Filter/1(In1)
  Demux/2 -> Analog Butterworth LP Filter1/1(In1)

== system Copy_3_of_proba1_poziomywsk/serwomechanizmy/os5/Position 5/Position Calculation 5 ==
  Sin : Inport
  Cos : Inport  Port=2
  Reset (Impulse) : Inport  Port=3
  Atan2 : Fcn  Expr=atan2(u[1],u[2])
  Conversion Rad to Deg : Gain  Gain=180/pi  SaturateOnIntegerOverflow=on
  Conversion Rotation to Angle : Gain  Gain=2*pi  SaturateOnIntegerOverflow=on
  Dead Zone : DeadZone  LowerValue=-5000  UpperValue=5000  SaturateOnIntegerOverflow=on
  Derivative : Derivative
  Gear : Gain  Gain=1.32e-2  SaturateOnIntegerOverflow=on
  Init Angle : Switch  Threshold=1  SaturateOnIntegerOverflow=on  InputSameDT=on
  Memory : Memory  Orientation=left
  Memory1 : Memory  Orientation=left
  Mux : Mux  Inputs=2
  Product : Product  SaturateOnIntegerOverflow=on  RndMeth=Zero  InputSameDT=on
  Saturation : Saturate  UpperLimit=1  LowerLimit=-1
  Sum : Sum  Inputs=+-  SaturateOnIntegerOverflow=on  InputSameDT=on
  Sum1 : Sum  Inputs=++-  SaturateOnIntegerOverflow=on  InputSameDT=on
  Position : Outport
  wires:
  Gear/1 -> Conversion Rad to Deg/1
  Sum1/1 -> Gear/1
  Sum/1 -> Product/1
  Dead Zone/1 -> Saturation/1
  Derivative/1 -> Dead Zone/1
  Mux/1 -> Atan2/1
  Sin/1 -> Mux/1
  Conversion Rad to Deg/1 -> Position/1
  Saturation/1 -> Sum/2
  Conversion Rotation to Angle/1 -> Sum1/1
  Reset (Impulse)/1 -> Product/2, Init Angle/2
  Atan2/1 -> Derivative/1, Sum1/2, Init Angle/3
  Cos/1 -> Mux/2
  Memory/1 -> Sum/1
  Product/1 -> Conversion Rotation to Angle/1, Memory/1
  Memory1/1 -> Init Angle/1
  Init Angle/1 -> Sum1/3, Memory1/1

== system Copy_3_of_proba1_poziomywsk/serwomechanizmy/os5/blok bazowania/zerowanie ==
  Enable : EnablePort
  Constant : Constant  Value=0
  Data Store Write : DataStoreWrite  DataStoreName=u5  SampleTime=-1
  Data Store Write1 : DataStoreWrite  DataStoreName=tmp_u5  SampleTime=-1
  wires:
  Constant/1 -> Data Store Write/1, Data Store Write1/1

== system Copy_3_of_proba1_poziomywsk/serwomechanizmy/os6/blok bazowania/zerowanie ==
  Enable : EnablePort
  Constant : Constant  Value=0
  Data Store Write : DataStoreWrite  DataStoreName=u0  SampleTime=-1
  Data Store Write1 : DataStoreWrite  DataStoreName=tmp_u0  SampleTime=-1
  wires:
  Constant/1 -> Data Store Write/1, Data Store Write1/1

== system Copy_3_of_proba1_poziomywsk/tryby/kinematyka odwrotna/optymalizacja1/warunek na Fi ==
  In2 : Inport
  warunek : Inport  Port=2
  FImax : Constant  Value=8*pi()/9  OutDataTypeMode=double
      settings: SamplingMode=Frame based
  FImin1 : Constant  Value=-8*pi()/9  OutDataTypeMode=double
      settings: SamplingMode=Frame based
  Mux1 : Mux  Inputs=2
  Mux3 : Mux  Inputs=2
  Subsystem1 : Subsystem
  Subsystem4 : Subsystem
  Switch1 : Switch  Criteria=u2 ~= 0  OutDataTypeMode=double
  Switch4 : Switch  Criteria=u2 ~= 0
  Switch5 : Switch  Criteria=u2 ~= 0
  Xgran : Fcn  Expr=u(1)*tan(u(4))
  Xnastawy1 : Fcn  Expr=u(2) - u(4)
  Xnastawy2 : Fcn  Expr=u(2) + u(4)
  nieosiagalna : Constant  Value=0  OutDataTypeMode=double
  Ynastawy : Outport
  wires:
  Xgran/1 -> Mux3/2
  FImax/1 -> Switch1/1
  Mux1/1 -> Xgran/1
  Mux3/1 -> Xnastawy1/1, Xnastawy2/1
  Subsystem4/1(Out1) -> Switch4/2
  Switch5/1 -> Switch4/3
  Subsystem1/1(Out1) -> Switch5/2
  nieosiagalna/1 -> Switch5/3
  Switch4/1 -> Ynastawy/1
  Xnastawy1/1 -> Subsystem4/1(In1), Switch4/1
  Xnastawy2/1 -> Switch5/1, Subsystem1/1(In1)
  In2/1 -> Mux1/1, Mux3/1
  Switch1/1 -> Mux1/2
  warunek/1 -> Switch1/2
  FImin1/1 -> Switch1/3

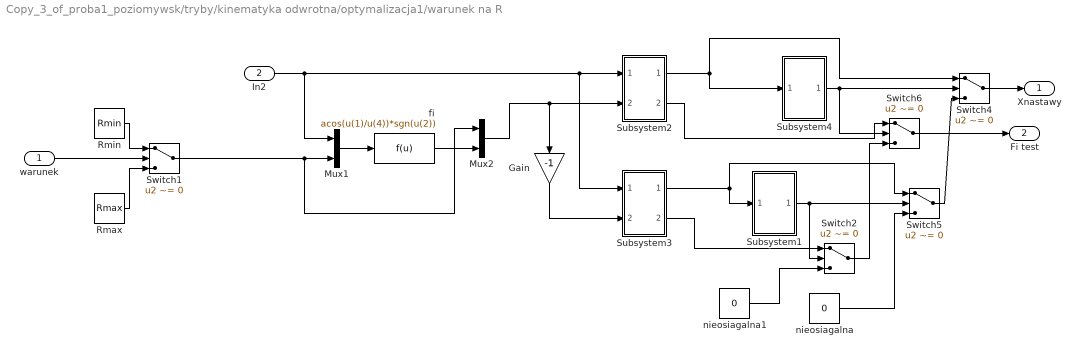
== system Copy_3_of_proba1_poziomywsk/tryby/kinematyka odwrotna/optymalizacja1/warunek na R ==
  warunek : Inport
  In2 : Inport  Port=2
  Gain : Gain  Orientation=down  Gain=-1
  Mux1 : Mux  Inputs=2
  Mux2 : Mux  Inputs=2
  Rmax : Constant  Value=Rmax  OutDataTypeMode=double
  Rmin : Constant  Value=Rmin  OutDataTypeMode=double
  Subsystem1 : Subsystem
  Subsystem2 : Subsystem
  Subsystem3 : Subsystem
  Subsystem4 : Subsystem
  Switch{1..2,4..6} (5 alike) : Switch  Criteria=u2 ~= 0
  fi : Fcn  Expr=acos(u(1)/u(4))*sgn(u(2))
  nieosiagalna : Constant  Value=0  OutDataTypeMode=double
  nieosiagalna1 : Constant  Value=0  OutDataTypeMode=double
  Xnastawy : Outport
  Fi test : Outport  Port=2
  wires:
  fi/1 -> Mux2/2
  Mux1/1 -> fi/1
  In2/1 -> Subsystem3/1(In2), Subsystem2/1(In2), Mux1/1
  Switch1/1 -> Mux1/2, Mux2/1
  warunek/1 -> Switch1/2
  Subsystem4/1(Out1) -> Switch6/2, Switch4/2
  Switch5/1 -> Switch4/3
  Subsystem1/1(Out1) -> Switch2/2, Switch5/2
  nieosiagalna/1 -> Switch5/3
  Mux2/1 -> Subsystem2/2(In3), Gain/1
  Switch6/1 -> Fi test/1
  Switch4/1 -> Xnastawy/1
  Gain/1 -> Subsystem3/2(In3)
  Subsystem3/1(Out1) -> Switch5/1, Subsystem1/1(In1)
  Subsystem3/2(Out2) -> Switch2/1
  Subsystem2/1(Out1) -> Subsystem4/1(In1), Switch4/1
  Subsystem2/2(Out2) -> Switch6/1
  Switch2/1 -> Switch6/3
  nieosiagalna1/1 -> Switch2/3
  Rmin/1 -> Switch1/1
  Rmax/1 -> Switch1/3

== system Copy_3_of_proba1_poziomywsk/tryby/rozpoznawanie obrazu/optymalizacja1/warunek na Fi ==
  In2 : Inport
  warunek : Inport  Port=2
  FImax : Constant  Value=8*pi()/9  OutDataTypeMode=double
      settings: SamplingMode=Frame based
  FImin1 : Constant  Value=-8*pi()/9  OutDataTypeMode=double
      settings: SamplingMode=Frame based
  Mux1 : Mux  Inputs=2
  Mux3 : Mux  Inputs=2
  Subsystem1 : Subsystem
  Subsystem4 : Subsystem
  Switch1 : Switch  Criteria=u2 ~= 0  OutDataTypeMode=double
  Switch4 : Switch  Criteria=u2 ~= 0
  Switch5 : Switch  Criteria=u2 ~= 0
  Xgran : Fcn  Expr=u(1)*tan(u(4))
  Xnastawy1 : Fcn  Expr=u(2) - u(4)
  Xnastawy2 : Fcn  Expr=u(2) + u(4)
  nieosiagalna : Constant  Value=0  OutDataTypeMode=double
  Ynastawy : Outport
  wires:
  FImin1/1 -> Switch1/3
  warunek/1 -> Switch1/2
  Switch1/1 -> Mux1/2
  In2/1 -> Mux3/1, Mux1/1
  Xnastawy2/1 -> Subsystem1/1(In1), Switch5/1
  Xnastawy1/1 -> Switch4/1, Subsystem4/1(In1)
  Switch4/1 -> Ynastawy/1
  nieosiagalna/1 -> Switch5/3
  Subsystem1/1(Out1) -> Switch5/2
  Switch5/1 -> Switch4/3
  Subsystem4/1(Out1) -> Switch4/2
  Mux3/1 -> Xnastawy2/1, Xnastawy1/1
  Mux1/1 -> Xgran/1
  FImax/1 -> Switch1/1
  Xgran/1 -> Mux3/2

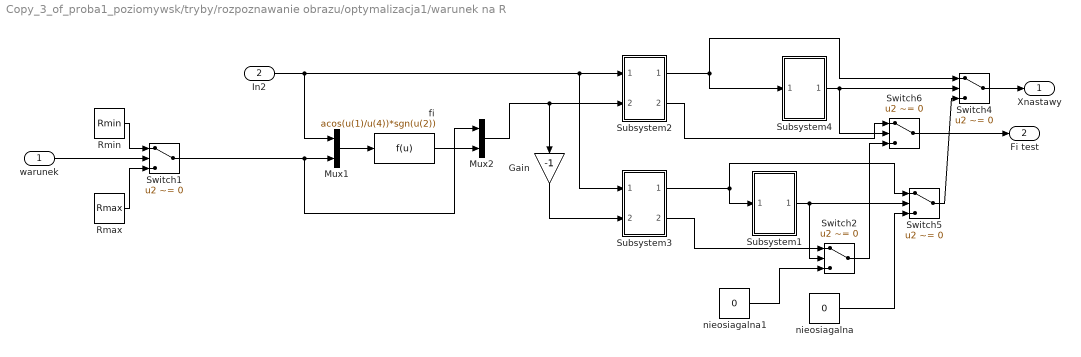
== system Copy_3_of_proba1_poziomywsk/tryby/rozpoznawanie obrazu/optymalizacja1/warunek na R ==
  warunek : Inport
  In2 : Inport  Port=2
  Gain : Gain  Orientation=down  Gain=-1
  Mux1 : Mux  Inputs=2
  Mux2 : Mux  Inputs=2
  Rmax : Constant  Value=Rmax  OutDataTypeMode=double
  Rmin : Constant  Value=Rmin  OutDataTypeMode=double
  Subsystem1 : Subsystem
  Subsystem2 : Subsystem
  Subsystem3 : Subsystem
  Subsystem4 : Subsystem
  Switch{1..2,4..6} (5 alike) : Switch  Criteria=u2 ~= 0
  fi : Fcn  Expr=acos(u(1)/u(4))*sgn(u(2))
  nieosiagalna : Constant  Value=0  OutDataTypeMode=double
  nieosiagalna1 : Constant  Value=0  OutDataTypeMode=double
  Xnastawy : Outport
  Fi test : Outport  Port=2
  wires:
  Rmax/1 -> Switch1/3
  Rmin/1 -> Switch1/1
  nieosiagalna1/1 -> Switch2/3
  Switch2/1 -> Switch6/3
  Subsystem2/2(Out2) -> Switch6/1
  Subsystem2/1(Out1) -> Switch4/1, Subsystem4/1(In1)
  Subsystem3/2(Out2) -> Switch2/1
  Subsystem3/1(Out1) -> Subsystem1/1(In1), Switch5/1
  Gain/1 -> Subsystem3/2(In3)
  Switch4/1 -> Xnastawy/1
  Switch6/1 -> Fi test/1
  Mux2/1 -> Gain/1, Subsystem2/2(In3)
  nieosiagalna/1 -> Switch5/3
  Subsystem1/1(Out1) -> Switch5/2, Switch2/2
  Switch5/1 -> Switch4/3
  Subsystem4/1(Out1) -> Switch4/2, Switch6/2
  warunek/1 -> Switch1/2
  Switch1/1 -> Mux2/1, Mux1/2
  In2/1 -> Mux1/1, Subsystem2/1(In2), Subsystem3/1(In2)
  Mux1/1 -> fi/1
  fi/1 -> Mux2/2

== system Copy_3_of_proba1_poziomywsk/RTI Data/RTI Data Store/RTI Data Store/RTI Data Store/RTI Data Store ==

== system Copy_3_of_proba1_poziomywsk/serwomechanizmy/os1/Position 1/Filters 1/Analog Butterworth LP Filter ==
  In1 : Inport
  Analog Butterworth LP Filter : ZeroPole  Zeros=z  Poles=p  Gain=k
  Out1 : Outport
  wires:
  Analog Butterworth LP Filter/1 -> Out1/1
  In1/1 -> Analog Butterworth LP Filter/1

== system Copy_3_of_proba1_poziomywsk/serwomechanizmy/os1/Position 1/Filters 1/Analog Butterworth LP Filter1 ==
  In1 : Inport
  Analog Butterworth LP Filter1 : ZeroPole  Zeros=z  Poles=p  Gain=k
  Out1 : Outport
  wires:
  Analog Butterworth LP Filter1/1 -> Out1/1
  In1/1 -> Analog Butterworth LP Filter1/1

== system Copy_3_of_proba1_poziomywsk/serwomechanizmy/os2/Position 2/Filters 2/Analog Butterworth LP Filter ==
  In1 : Inport
  Analog Butterworth LP Filter : ZeroPole  Zeros=z  Poles=p  Gain=k
  Out1 : Outport
  wires:
  Analog Butterworth LP Filter/1 -> Out1/1
  In1/1 -> Analog Butterworth LP Filter/1

== system Copy_3_of_proba1_poziomywsk/serwomechanizmy/os2/Position 2/Filters 2/Analog Butterworth LP Filter1 ==
  In1 : Inport
  Analog Butterworth LP Filter1 : ZeroPole  Zeros=z  Poles=p  Gain=k
  Out1 : Outport
  wires:
  Analog Butterworth LP Filter1/1 -> Out1/1
  In1/1 -> Analog Butterworth LP Filter1/1

== system Copy_3_of_proba1_poziomywsk/serwomechanizmy/os3/Position 3/Filters 3/Analog Butterworth LP Filter ==
  In1 : Inport
  Analog Butterworth LP Filter : ZeroPole  Zeros=z  Poles=p  Gain=k
  Out1 : Outport
  wires:
  Analog Butterworth LP Filter/1 -> Out1/1
  In1/1 -> Analog Butterworth LP Filter/1

== system Copy_3_of_proba1_poziomywsk/serwomechanizmy/os3/Position 3/Filters 3/Analog Butterworth LP Filter1 ==
  In1 : Inport
  Analog Butterworth LP Filter1 : ZeroPole  Zeros=z  Poles=p  Gain=k
  Out1 : Outport
  wires:
  Analog Butterworth LP Filter1/1 -> Out1/1
  In1/1 -> Analog Butterworth LP Filter1/1

== system Copy_3_of_proba1_poziomywsk/serwomechanizmy/os4/Position 4/Filters 4/Analog Butterworth LP Filter ==
  In1 : Inport
  Analog Butterworth LP Filter : ZeroPole  Zeros=z  Poles=p  Gain=k
  Out1 : Outport
  wires:
  Analog Butterworth LP Filter/1 -> Out1/1
  In1/1 -> Analog Butterworth LP Filter/1

== system Copy_3_of_proba1_poziomywsk/serwomechanizmy/os4/Position 4/Filters 4/Analog Butterworth LP Filter1 ==
  In1 : Inport
  Analog Butterworth LP Filter1 : ZeroPole  Zeros=z  Poles=p  Gain=k
  Out1 : Outport
  wires:
  Analog Butterworth LP Filter1/1 -> Out1/1
  In1/1 -> Analog Butterworth LP Filter1/1

== system Copy_3_of_proba1_poziomywsk/serwomechanizmy/os5/Position 5/Filters 5/Analog Butterworth LP Filter ==
  In1 : Inport
  Analog Butterworth LP Filter : ZeroPole  Zeros=z  Poles=p  Gain=k
  Out1 : Outport
  wires:
  Analog Butterworth LP Filter/1 -> Out1/1
  In1/1 -> Analog Butterworth LP Filter/1

== system Copy_3_of_proba1_poziomywsk/serwomechanizmy/os5/Position 5/Filters 5/Analog Butterworth LP Filter1 ==
  In1 : Inport
  Analog Butterworth LP Filter1 : ZeroPole  Zeros=z  Poles=p  Gain=k
  Out1 : Outport
  wires:
  Analog Butterworth LP Filter1/1 -> Out1/1
  In1/1 -> Analog Butterworth LP Filter1/1

== system Copy_3_of_proba1_poziomywsk/tryby/kinematyka odwrotna/optymalizacja1/warunek na Fi/Subsystem1 ==
  In1 : Inport
  Add : Sum  Inputs=++|
  Data Store Read6 : DataStoreRead  DataStoreName=yKon  SampleTime=0
  Logical Operator4 : Logic  AllPortsSameDT=off  OutDataTypeMode=boolean
  do Xmax : simulink/Logic and Bit Operations/Compare To Constant  SystemSampleTime=-1  relop=<  const=1600  LogicOutDataTypeMode=uint8  ZeroCross=off
  do Xmin : simulink/Logic and Bit Operations/Compare To Constant  SystemSampleTime=-1  relop=>  const=0  LogicOutDataTypeMode=uint8  ZeroCross=off
  Out1 : Outport
  wires:
  In1/1 -> Add/1
  Logical Operator4/1 -> Out1/1
  Add/1 -> do Xmax/1, do Xmin/1
  do Xmax/1 -> Logical Operator4/2
  do Xmin/1 -> Logical Operator4/1
  Data Store Read6/1 -> Add/2

== system Copy_3_of_proba1_poziomywsk/tryby/kinematyka odwrotna/optymalizacja1/warunek na Fi/Subsystem4 ==
  In1 : Inport
  Add : Sum  Inputs=++|
  Data Store Read6 : DataStoreRead  DataStoreName=yKon  SampleTime=0
  Logical Operator4 : Logic  AllPortsSameDT=off  OutDataTypeMode=boolean
  do Xmax : simulink/Logic and Bit Operations/Compare To Constant  SystemSampleTime=-1  relop=<  const=1600  LogicOutDataTypeMode=uint8  ZeroCross=off
  do Xmin : simulink/Logic and Bit Operations/Compare To Constant  SystemSampleTime=-1  relop=>  const=0  LogicOutDataTypeMode=uint8  ZeroCross=off
  Out1 : Outport
  wires:
  do Xmin/1 -> Logical Operator4/1
  do Xmax/1 -> Logical Operator4/2
  Data Store Read6/1 -> Add/2
  Add/1 -> do Xmin/1, do Xmax/1
  Logical Operator4/1 -> Out1/1
  In1/1 -> Add/1

== system Copy_3_of_proba1_poziomywsk/tryby/kinematyka odwrotna/optymalizacja1/warunek na R/Subsystem1 ==
  In1 : Inport
  Add : Sum  Inputs=++|
  Data Store Read6 : DataStoreRead  DataStoreName=yKon  SampleTime=0
  Logical Operator4 : Logic  AllPortsSameDT=off  OutDataTypeMode=boolean
  do Xmax : simulink/Logic and Bit Operations/Compare To Constant  SystemSampleTime=-1  relop=<  const=1600  LogicOutDataTypeMode=uint8  ZeroCross=off
  do Xmin : simulink/Logic and Bit Operations/Compare To Constant  SystemSampleTime=-1  relop=>  const=0  LogicOutDataTypeMode=uint8  ZeroCross=off
  Out1 : Outport
  wires:
  In1/1 -> Add/1
  Logical Operator4/1 -> Out1/1
  Add/1 -> do Xmax/1, do Xmin/1
  do Xmax/1 -> Logical Operator4/2
  do Xmin/1 -> Logical Operator4/1
  Data Store Read6/1 -> Add/2
